simulink library "manualMotorOverride"  (R2018b)
settings: Solver=VariableStepAuto  StartTime=0.0  StopTime=10.0  RelTol=1e-3
settings Model: Creator=mcobb  LastModifiedBy=mcobb

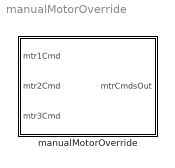
== system manualMotorOverride ==
  manualMotorOverride : Subsystem  mask{enbl=0, mtr1CmdOvrrd=0, mtr2CmdOvrrd=0, mtr3CmdOvrrd=0}
      mask prompts: enbl "Control Mode (0 = manual, 1 = Auto)"; mtr1CmdOvrrd "Motor 1 Override Command [-1 1]"; mtr2CmdOvrrd "Motor 2 Override Command [-1 1]"; mtr3CmdOvrrd "Motor 3 Override Command [-1 1]"
      mask Display:
      | enbl = get_param(gcb,'enbl');
      | 
      | if strcmpi(enbl,0)
      | %     color = [0 0.7 0];
      |     str = 'MANUAL';
      | else
      | %     color = [0.7 0 0];
      |     str = 'AUTOMATIC';
      | end
      | % patch([0.25 0.75 0.75 0.25], [0.8 0.8 1 1],color)
      | 
      | text(0.5, 0.85, str, 'horizontalAlignment', 'center','verticalAlignment','bottom')
      | port_label('input',1,'mtr1Cmd')
      | port_label('input',2,'mtr2Cmd')
      | port_label('input',3,'mtr3Cmd')
      | port_label('output',1,'mtrCmds')
      | 
      | % port_label('output',1,'motorVoltages_V')
      | % port_label('output',2,'motorVoltages_V')

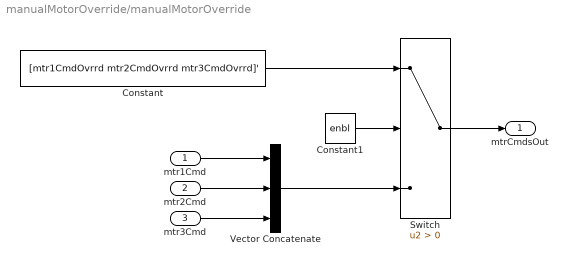
== system manualMotorOverride/manualMotorOverride ==
  mtr1Cmd : Inport
  mtr2Cmd : Inport  Port=2
  mtr3Cmd : Inport  Port=3
  Constant : Constant  Value=[mtr1CmdOvrrd mtr2CmdOvrrd mtr3CmdOvrrd]'
  Constant1 : Constant  Value=enbl
  Switch : Switch  Criteria=u2 > Threshold
  Vector Concatenate : Concatenate  NumInputs=3
  mtrCmdsOut : Outport
  wires:
  Constant/1 -> Switch/1
  Constant1/1 -> Switch/2
  Switch/1 -> mtrCmdsOut/1
  Vector Concatenate/1 -> Switch/3
  mtr1Cmd/1 -> Vector Concatenate/1
  mtr2Cmd/1 -> Vector Concatenate/2
  mtr3Cmd/1 -> Vector Concatenate/3
